simulink model "debugread"  (R2024b)
settings: Solver=VariableStepAuto  StartTime=0.0  StopTime=inf  RelTol=1e-3
settings Model: Creator=kev  LastModifiedBy=kev

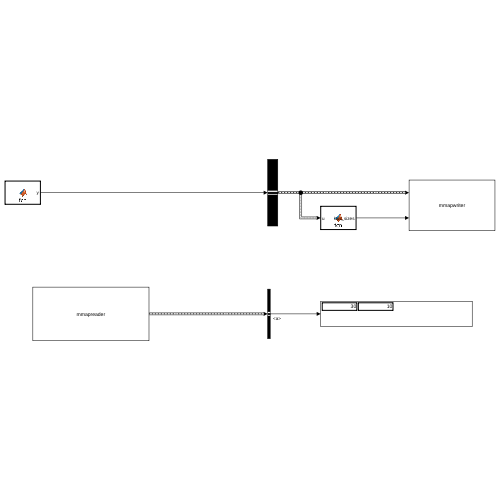
[thumbnail: Simulink's stored preview of the top-level diagram]
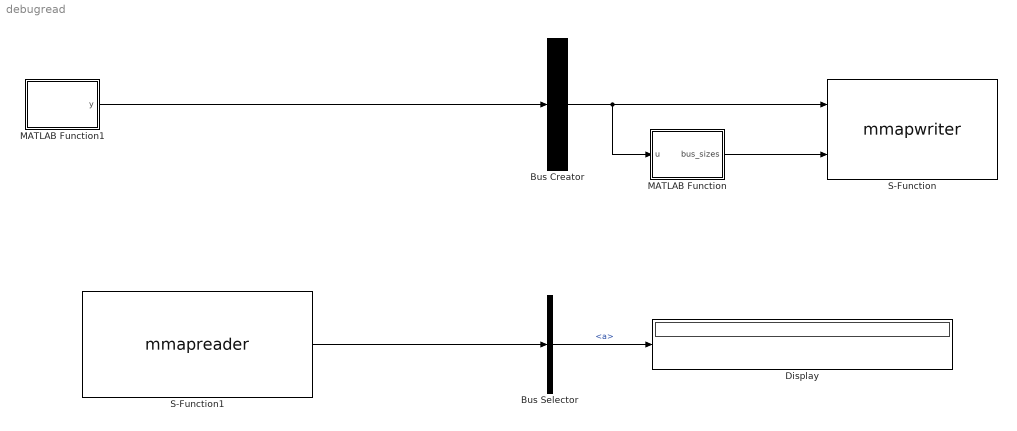
== system debugread ==
  Bus Creator : BusCreator  Inputs=1  OutDataTypeStr=Bus: TestBus  NonVirtualBus=on
      settings: InheritFromInputs=off
  Bus Selector : BusSelector  OutputSignals=a
  Display : Display
  MATLAB Function : MATLAB Function  TreatAsAtomicUnit=on
  MATLAB Function1 : MATLAB Function  TreatAsAtomicUnit=on
  S-Function : S-Function  FunctionName=mmapwriter  Parameters=TestBus, 'TestingBus'  SFunctionDeploymentMode=off  EnableBusSupport=off
  S-Function1 : S-Function  FunctionName=mmapreader  Parameters='TestingBus', TestBus  SFunctionDeploymentMode=off  EnableBusSupport=off
  wires:
  MATLAB Function1/1(y) -> Bus Creator/1
  Bus Creator/1 -> MATLAB Function/1(u), S-Function/1
  MATLAB Function/1(bus_sizes) -> S-Function/2
  S-Function1/1 -> Bus Selector/1
  Bus Selector/1 -> Display/1  "<a>"

== matlab function debugread/MATLAB Function ==
  data: u input; bus_sizes output
function bus_sizes   = fcn(u)
    flat_dims = zeros(getLen(u), 2, 'int32');
    counter = ones(1);
    [flat_dims, counter] = getDims(u, flat_dims, counter);
    bus_sizes = flat_dims;
    %disp(flat_dims);
end

function len = getLen(bus)
    fields = fieldnames(bus);
    len = 0;
    for iF = 1:numel(fields)
        field = fields{iF};
        if isfield(bus, field)
            value = bus.(field);
            if isa(value, 'struct')
                len = len + getLen(value);
            else
                len = len + 1;
            end
        end
    end
end

function [flat_dims, counter] = getDims(bus, flat_dims, counter)
    fields = fieldnames(bus);
    for iF = 1:numel(fields)
        field = fields{iF};
        if isfield(bus, field)
            value = bus.(field);
            if isa(value, 'struct')
                [flat_dims, counter] = getDims(value, flat_dims, counter);
            else
                flat_dims(counter(1), :) = size(value);
                counter(1) = counter(1) + 1;
            end
        end
    end
end

== matlab function debugread/MATLAB Function1 ==
  data: y output size=2
function y = fcn()
    y = [3; 1];
end
